simulink model "mut_duty_cycle_waveform_generator"  (R2020b)
settings: Solver=FixedStepAuto  StartTime=0.0  StopTime=10.0  FixedStep=6.25e-6  RelTol=1e-3
libraries: vhit_control_library x1
settings Model: DataDictionary=dd_model_under_test_data.sldd  EnableAccessToBaseWorkspace=off  Creator=CAV2OFO  LastModifiedBy=CAV2OFO
settings DebuggingCC: ParameterPrecisionLossMsg=none

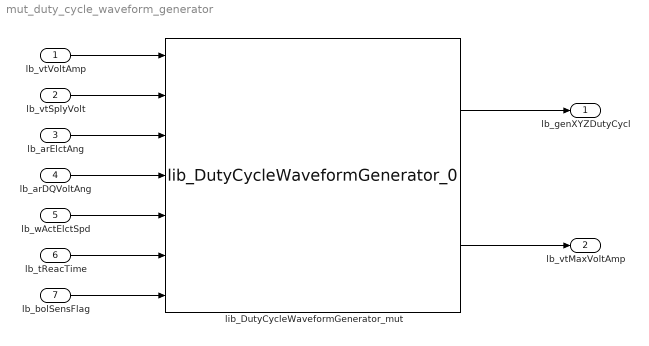
== system mut_duty_cycle_waveform_generator ==
  lb_vtVoltAmp : Inport  OutDataTypeStr=fixdt(1,16,2^-9,0)  Interpolate=off
  lb_vtSplyVolt : Inport  Port=2  OutDataTypeStr=fixdt(1,16,2^-9,0)  Interpolate=off
  lb_arElctAng : Inport  Port=3  OutDataTypeStr=fixdt(0,16,pi*2^-15,0)  Interpolate=off
  lb_arDQVoltAng : Inport  Port=4  OutDataTypeStr=fixdt(0,16,pi*2^-15,0)  Interpolate=off
  lb_wActElctSpd : Inport  Port=5  OutDataTypeStr=fixdt(1,16,2^-3,0)  Interpolate=off
  lb_tReacTime : Inport  Port=6  OutDataTypeStr=fixdt(0,16,2^-26,0)  Interpolate=off
  lb_bolSensFlag : Inport  Port=7  OutDataTypeStr=boolean
  lib_DutyCycleWaveformGenerator_mut : vhit_control_library/lib_DutyCycleWaveformGenerator_0  lb_parLktSize=1024  lb_parOmodFact=parOmodFact  lb_parPWMMode=Discontinuous minimum modulation  lb_parSimModeFlag=off
  lb_genXYZDutyCycl : Outport  OutDataTypeStr=fixdt(0,16,2^-15,0)
  lb_vtMaxVoltAmp : Outport  Port=2
  wires:
  lib_DutyCycleWaveformGenerator_mut/1 -> lb_genXYZDutyCycl/1
  lb_vtVoltAmp/1 -> lib_DutyCycleWaveformGenerator_mut/1
  lib_DutyCycleWaveformGenerator_mut/2 -> lb_vtMaxVoltAmp/1
  lb_vtSplyVolt/1 -> lib_DutyCycleWaveformGenerator_mut/2
  lb_arElctAng/1 -> lib_DutyCycleWaveformGenerator_mut/3
  lb_arDQVoltAng/1 -> lib_DutyCycleWaveformGenerator_mut/4
  lb_wActElctSpd/1 -> lib_DutyCycleWaveformGenerator_mut/5
  lb_tReacTime/1 -> lib_DutyCycleWaveformGenerator_mut/6
  lb_bolSensFlag/1 -> lib_DutyCycleWaveformGenerator_mut/7
